simulink subsystem "RackAndPinion"  (R2022b)
settings: Solver=VariableStepAuto  StartTime=0.0  StopTime=10.0  RelTol=1e-3
undefined symbols (not defined in the file): ProjectExample
settings Model: Creator=Ilya_Andriyanov  LastModifiedBy=user

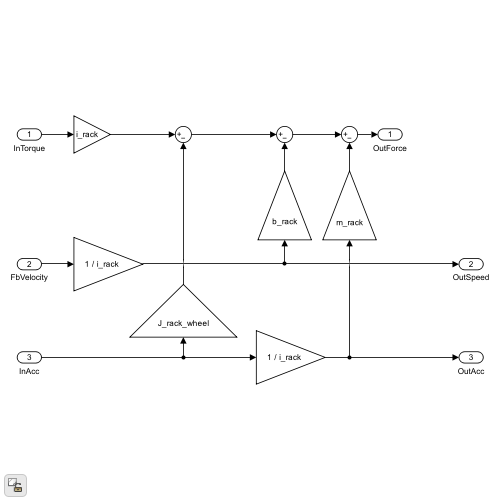
[thumbnail: Simulink's stored preview of the top-level diagram]
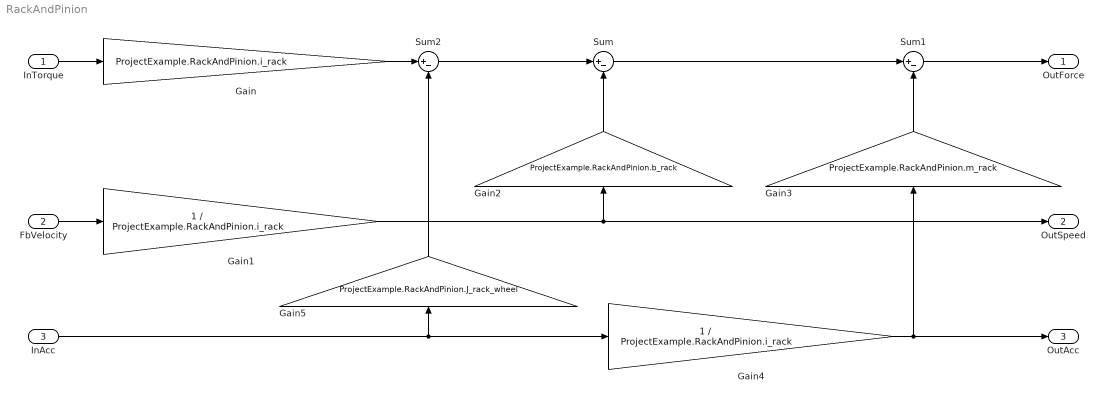
== system RackAndPinion ==
  InTorque : Inport
  FbVelocity : Inport  Port=2
  InAcc : Inport  Port=3
  Gain : Gain  Gain=ProjectExample.RackAndPinion.i_rack
  Gain1 : Gain  Gain=1 / ProjectExample.RackAndPinion.i_rack
  Gain2 : Gain  Gain=ProjectExample.RackAndPinion.b_rack
  Gain3 : Gain  Gain=ProjectExample.RackAndPinion.m_rack
  Gain4 : Gain  Gain=1 / ProjectExample.RackAndPinion.i_rack
  Gain5 : Gain  Gain=ProjectExample.RackAndPinion.J_rack_wheel
  Sum : Sum  Inputs=|+-
  Sum1 : Sum  Inputs=|+-
  Sum2 : Sum  Inputs=|+-
  OutForce : Outport
  OutSpeed : Outport  Port=2
  OutAcc : Outport  Port=3
  wires:
  Gain3/1 -> Sum1/2
  InAcc/1 -> Gain5/1, Gain4/1
  Gain2/1 -> Sum/2
  Gain1/1 -> Gain2/1, OutSpeed/1
  Sum/1 -> Sum1/1
  Sum1/1 -> OutForce/1
  InTorque/1 -> Gain/1
  FbVelocity/1 -> Gain1/1
  Gain4/1 -> Gain3/1, OutAcc/1
  Sum2/1 -> Sum/1
  Gain/1 -> Sum2/1
  Gain5/1 -> Sum2/2
